simulink model "AP2_discret_sim"  (R2022b)
settings: Solver=VariableStepAuto  StartTime=0.0  StopTime=10  RelTol=1e-3
values from neighbouring files (symbols this model uses):
  denGz_1 = cell2mat(Gz_1.Denominator)    [Ap1_Ap2.m]
  denGz_2 = cell2mat(Gz_2.Denominator)    [Ap1_Ap2.m]
  denGz_3 = cell2mat(Gz_3.Denominator)    [Ap1_Ap2.m]
  denRz_1 = cell2mat(Rz_1.Denominator)    [Ap1_Ap2.m]
  denRz_2 = cell2mat(Rz_2.Denominator)    [Ap1_Ap2.m]
  denRz_3 = cell2mat(Rz_3.Denominator)    [Ap1_Ap2.m]
  numGz_1 = cell2mat(Gz_1.Numerator)    [Ap1_Ap2.m]
  numGz_2 = cell2mat(Gz_2.Numerator)    [Ap1_Ap2.m]
  numGz_3 = cell2mat(Gz_3.Numerator)    [Ap1_Ap2.m]
  numRz_1 = cell2mat(Rz_1.Numerator)    [Ap1_Ap2.m]
  numRz_2 = cell2mat(Rz_2.Numerator)    [Ap1_Ap2.m]
  numRz_3 = cell2mat(Rz_3.Numerator)    [Ap1_Ap2.m]
libraries: simulink x1
settings Model: Creator=mluser  LastModifiedBy=mluser

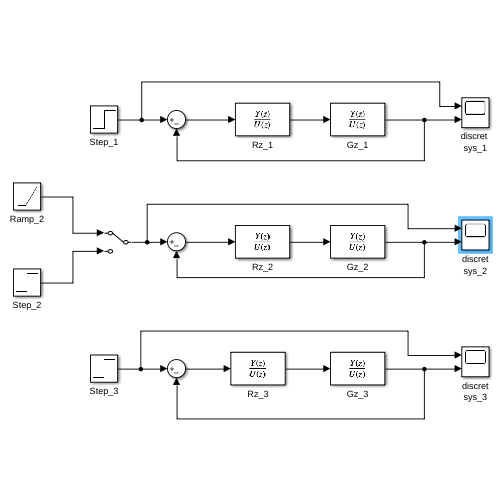
[thumbnail: Simulink's stored preview of the top-level diagram]
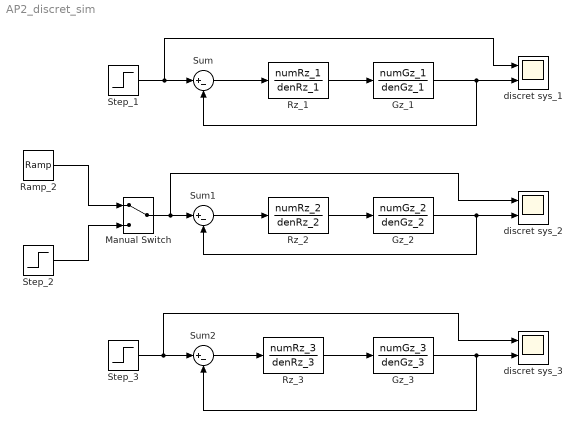
== system AP2_discret_sim ==
  Gz_1 : DiscreteTransferFcn  Numerator=numGz_1  Denominator=denGz_1
  Gz_2 : DiscreteTransferFcn  Numerator=numGz_2  Denominator=denGz_2
  Gz_3 : DiscreteTransferFcn  Numerator=numGz_3  Denominator=denGz_3
  Manual Switch : ManualSwitch
  Ramp_2 : simulink/Sources/Ramp  slope=1  start=0  InitialOutput=0
  Rz_1 : DiscreteTransferFcn  Numerator=numRz_1  Denominator=denRz_1
  Rz_2 : DiscreteTransferFcn  Numerator=numRz_2  Denominator=denRz_2
  Rz_3 : DiscreteTransferFcn  Numerator=numRz_3  Denominator=denRz_3
  Step_1 : Step  SampleTime=0
  Step_2 : Step  SampleTime=0
  Step_3 : Step  SampleTime=0
  Sum : Sum  Inputs=|+-
  Sum1 : Sum  Inputs=|+-
  Sum2 : Sum  Inputs=|+-
  discret sys_2 : Scope  NumInputPorts=2
  discret sys_3 : Scope  NumInputPorts=2
  discret sys_1 : Scope  NumInputPorts=2
  wires:
  Ramp_2/1 -> Manual Switch/1
  Step_3/1 -> discret sys_3/1, Sum2/1
  Step_2/1 -> Manual Switch/2
  Step_1/1 -> Sum/1, discret sys_1/1
  Manual Switch/1 -> discret sys_2/1, Sum1/1
  Sum/1 -> Rz_1/1
  Rz_1/1 -> Gz_1/1
  Gz_1/1 -> discret sys_1/2, Sum/2
  Sum1/1 -> Rz_2/1
  Rz_2/1 -> Gz_2/1
  Gz_2/1 -> Sum1/2, discret sys_2/2
  Gz_3/1 -> discret sys_3/2, Sum2/2
  Rz_3/1 -> Gz_3/1
  Sum2/1 -> Rz_3/1
